simulink model "Gravitationspendel"  (R2021b)
settings: Solver=ode45  StartTime=0.0  StopTime=150  MaxStep=0.1  RelTol=1e-3  EnableMultiTasking=on
values from neighbouring files (symbols this model uses):
  g = 9.81    [SimulationScriptGravitationspendel.m]
  l = 5    [SimulationScriptGravitationspendel.m]
  omega_0 = 0    [SimulationScriptGravitationspendel.m]
  phi_0 = 45    [SimulationScriptGravitationspendel.m]
settings Model: Creator=matsim  LastModifiedBy=michi
settings SolverCC: AlgebraicLoopSolver=TrustRegion
settings DataIOCC: LimitDataPoints=on  SaveFormat=Array  SignalLoggingSaveFormat=ModelDataLogs  ReturnWorkspaceOutputs=off
settings OptimizationCC: BlockReduction=off  OptimizeBlockIOStorage=off  BufferReuse=off  GlobalBufferReuse=off  ExpressionFolding=off  ExpressionDepthLimit=2147483647  LocalBlockOutputs=off  LifeSpan=inf
settings DebuggingCC: UnderspecifiedInitializationDetection=Classic  MergeDetectMultiDrivingBlocksExec=none  SolverPrmCheckMsg=warning  FcnCallInpInsideContextMsg=warning  StateNameClashWarn=warning  SFUnexpectedBacktrackingDiag=warning  SFNoUnconditionalDefaultTransitionDiag=warning  SFExecutionAtInitializationDiag=none  SFMachineParentedDataDiag=warning  ArithmeticOperatorsInVariantConditions=warning
settings HardwareCC: ProdBitPerPointer=32  ProdBitPerSizeT=32  ProdBitPerPtrDiffT=32  ProdLargestAtomicFloat=None  ProdIntDivRoundTo=Undefined  ProdEndianess=Unspecified  ProdWordSize=32  ProdHWDeviceType=32-bit Generic
settings ModelReferenceCC: PropagateSignalLabelsOutOfModel=off
settings SFSimCC: SimUseLocalCustomCode=off  CustomCodeUndefinedFunction=UseInterfaceOnly
settings RTWCC: RTWUseLocalCustomCode=off
settings CodeAppCC: StateflowObjectComments=on
settings GRTTargetCC: TargetLangStandard=C89/C90 (ANSI)  CombineOutputUpdateFcns=off  GRTInterface=on
settings ConfigComp: CovMetricSettings=dw  CovSaveCumulativeToWorkspaceVar=on  CovSaveSingleToWorkspaceVar=on  CovExternalEMLEnable=off

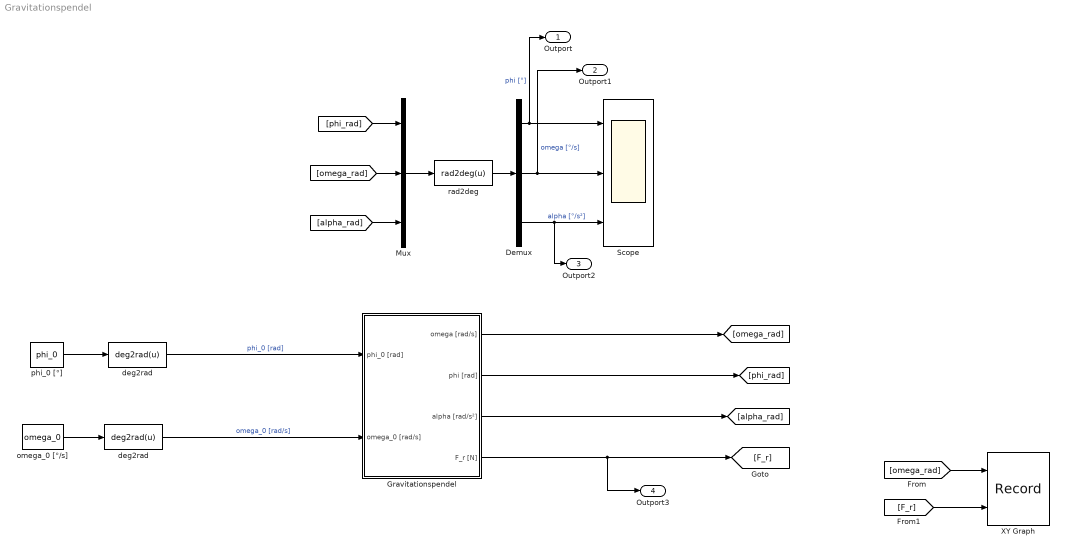
== system Gravitationspendel ==
  Demux : Demux  Outputs=3
  Gravitationspendel : Subsystem
  Mux : Mux  Inputs=3
  "Scope " : Scope  NumInputPorts=3
  XY Graph : Record  FileSettingsInternal="{\"entries\":[{\"content\":{\"excelSettings\":{\"content\":{},\"type\":\"Streamout.ExcelSettings\"}},\"type\":\"Streamout.FileSettingStorage\",\"uuid\":\"26158fd6-0bf1-434f-9cb4-7685c37aca91\"}],\"packageUris\":[\"http://schema.mathworks.com/mf0/streamout_blocks/R2020a\"],\"version\":\"1.0\"}"  Layout=[1 1]  SignalsInternal="{\"entries\":[{\"content\":{\"signals\":[{\"content\":{\"blockPath\":[\"Gravitationspendel/XY Graph\"],\"channel\":[],\"dimensions\":[1],\"domain\":\"Gravitationspendel/XY Graph\",\"lineColor\":\"#a2142f\",\"plots\":[1],\"port\":1,\"sid\":[],\"signalID\":9,\"signalName\":\"From\"},\"type\":\"RecordBlkView.Signal\",\"uuid\":\"f5222edd-907d-4328-85d2-7da264197bcc\"},{\"content\":{\"blockPath\":[\"Gravitationspendel/XY Graph\"],\"channel\":[],\"dimensions\":[1],\"domain\":\"Gravitationspendel/XY Graph\",\"lineColor\":\"#139fff\",\"plots\":[1],\"port\":2,\"sid\":[],\"signalID\":12,\"signalName\":\"From1\"},\"type\":\"RecordBlkView.Signal\",\"uuid\":\"761d0bc1-9f1f-4599-bf5b-d5aca5b2b02d\"}]},\"type\":\"RecordBlkView.InputSignals\",\"uuid\":\"f4e951d5-073c-4e04-af0f-7e16cd010dfa\"}],\"packageUris\":[\"http://schema.mathworks.com/mf0/streamout_blocks/R2020a\"],\"version\":\"1.0\"}"  VisualizationBindings="{\"xyplotplugin\":{\"info\":[{\"series\":[{\"bindingParametersList\":[{\"parameter\":\"X-Axis\",\"signalID\":9,\"signalName\":\"From\"},{\"parameter\":\"Y-Axis\",\"signalID\":12,\"signalName\":\"From1\"}],\"seriesID\":58936}],\"subplotID\":1}]}}"  CompatibilityTag=XY
  deg2rad : MATLABFcn  MATLABFcn=deg2rad(u)
  "deg2rad " : MATLABFcn  MATLABFcn=deg2rad(u)
  omega_0 [°/s] : Constant  Value=omega_0
  phi_0 [°] : Constant  Value=phi_0
  "rad2deg  " : MATLABFcn  MATLABFcn=rad2deg(u)
  Outport : Outport
  Outport1 : Outport  Port=2
  Outport2 : Outport  Port=3
  Outport3 : Outport  Port=4
  wires:
  Mux/1 -> "rad2deg  "/1
  "rad2deg  "/1 -> Demux/1
  Demux/3 -> Outport2/1, "Scope "/3  "alpha [°/s²]"
  Demux/2 -> Outport1/1, "Scope "/2  "omega [°/s]"
  Demux/1 -> "Scope "/1, Outport/1  "phi [°]"
  [phi_rad] -> Mux/1
  [omega_rad] -> Mux/2
  [alpha_rad] -> Mux/3
  [F_r] -> XY Graph/2
  [omega_rad] -> XY Graph/1
  phi_0 [°]/1 -> "deg2rad "/1
  omega_0 [°/s]/1 -> deg2rad/1
  "deg2rad "/1 -> Gravitationspendel/1(phi_0 [rad])  "phi_0 [rad]"
  deg2rad/1 -> Gravitationspendel/2(omega_0 [rad/s])  "omega_0 [rad/s]"
  Gravitationspendel/1(omega [rad/s]) -> [omega_rad]
  Gravitationspendel/2(phi [rad]) -> [phi_rad]
  Gravitationspendel/3(alpha [rad/s²]) -> [alpha_rad]
  Gravitationspendel/4(F_r [N]) -> Outport3/1, [F_r]

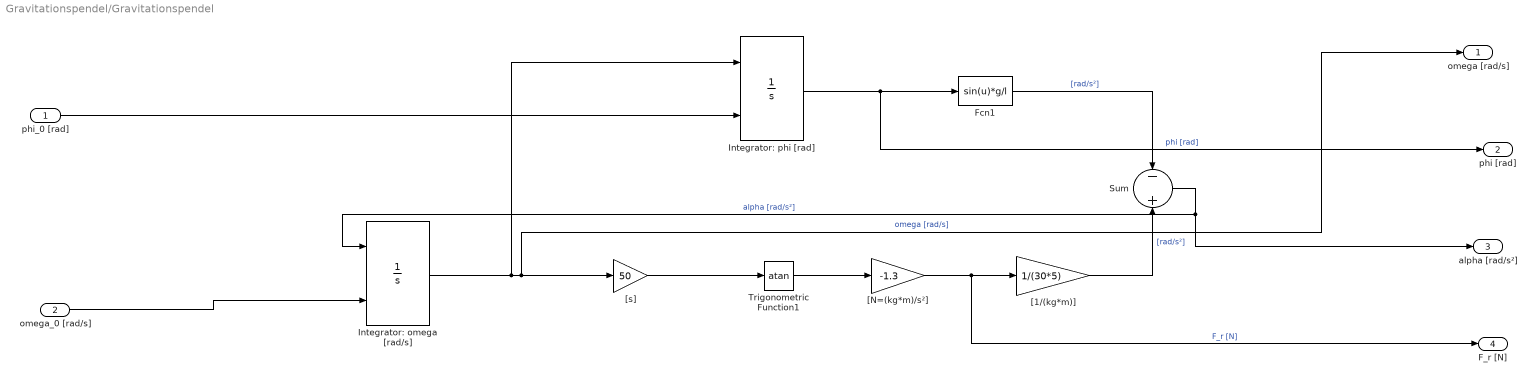
== system Gravitationspendel/Gravitationspendel ==
  phi_0 [rad] : Inport
  omega_0 [rad/s] : Inport  Port=2
  Fcn1 : Fcn  Expr=sin(u)*g/l
  Integrator: omega [rad/s] : Integrator  InitialConditionSource=external
  Integrator: phi [rad] : Integrator  InitialConditionSource=external
  Sum : Sum  Inputs=-|+
  Trigonometric Function1 : Trigonometry  Operator=atan
  "[1/(kg*m)]" : Gain  Gain=1/(30*5)
  "[N=(kg*m)/s²]" : Gain  Gain=-1.3
  "[s]" : Gain  Gain=50
  omega [rad/s] : Outport
  phi [rad] : Outport  Port=2
  alpha [rad/s²] : Outport  Port=3
  F_r [N] : Outport  Port=4
  wires:
  Sum/1 -> alpha [rad/s²]/1, Integrator: omega [rad/s]/1  "alpha [rad/s²]"
  "[s]"/1 -> Trigonometric Function1/1
  Integrator: omega [rad/s]/1 -> omega [rad/s]/1, "[s]"/1, Integrator: phi [rad]/1  "omega [rad/s]"
  Integrator: phi [rad]/1 -> phi [rad]/1, Fcn1/1  "phi [rad]"
  "[N=(kg*m)/s²]"/1 -> F_r [N]/1, "[1/(kg*m)]"/1  "F_r [N]"
  Fcn1/1 -> Sum/1  "[rad/s²]"
  Trigonometric Function1/1 -> "[N=(kg*m)/s²]"/1
  "[1/(kg*m)]"/1 -> Sum/2  "[rad/s²]"
  phi_0 [rad]/1 -> Integrator: phi [rad]/2
  omega_0 [rad/s]/1 -> Integrator: omega [rad/s]/2
